simulink model "Lab1_6A"  (R2018a)
settings: Solver=VariableStepAuto  StartTime=0.0  StopTime=90  RelTol=1e-3
settings Model: Creator=melab2  LastModifiedBy=rahul

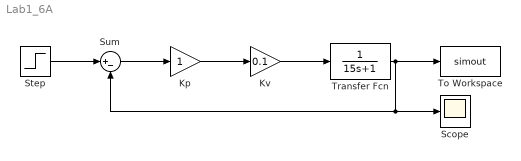
== system Lab1_6A ==
  Kp : Gain
  Kv : Gain  Gain=0.1
  Scope : Scope
  "Step " : Step  SampleTime=0
  Sum : Sum  Inputs=|+-
  To Workspace : ToWorkspace  VariableName=simout  SampleTime=-1
  Transfer Fcn : TransferFcn  Denominator=[15 1]
  wires:
  Sum/1 -> Kp/1
  "Step "/1 -> Sum/1
  Kp/1 -> Kv/1
  Kv/1 -> Transfer Fcn/1
  Transfer Fcn/1 -> Sum/2, Scope/1, To Workspace/1
